simulink model "MVC2025_sim"  (R2024b)
settings: Solver=FixedStepAuto  StartTime=0.0  StopTime=Tsim  FixedStep=Ts
InitFcn:
  | warning('off','all')
StopFcn:
  | warning('on','all')
undefined symbols (not defined in the file or in its folder): BAT, BUS, CTRLpmsm, CTRLtug, CTRLves, DiscIntNeverNeededParam, ESM, GEN, magnitude, MOT, RLgain, SM, tau0, Ts, TUG, VES
libraries: fl_lib x47, nesl_utility x35, simulink x24, slpidlib x10, ee_lib x10, sdl_lib x3, rllib x1, batteryecm_lib x1
(part 1 of 3)
settings Model: Creator=andreaturno  LastModifiedBy=sirpd
settings OptimizationCC: ReuseModelBlockBuffer=off
settings DebuggingCC: UnconnectedInputMsg=warning  UnconnectedOutputMsg=warning  UnconnectedLineMsg=warning
settings ModelReferenceCC: EnableRefExpFcnMdlSchedulingChecks=on
settings RTWCC: GPUComputeCapability=3.5  DLArmComputeVersion=19.05

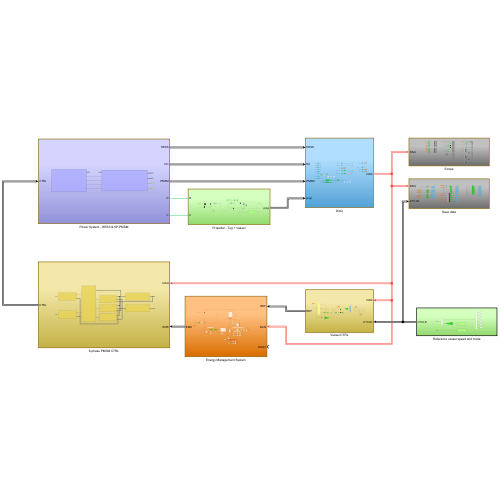
[thumbnail: Simulink's stored preview of the top-level diagram]
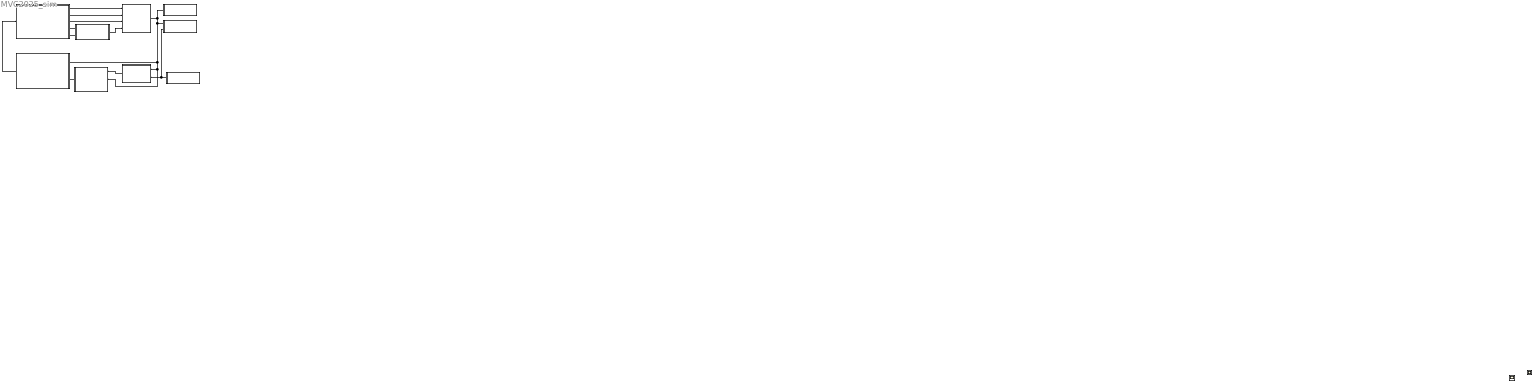
== system MVC2025_sim ==
  6-phase PMSM CTRL : Subsystem
  DAQ : Subsystem
  Energy Management System : Subsystem
  Power System - HESS & 6P-PMSM : Subsystem
  Propeller - Tug + Vessel : Subsystem
  Reference vessel speed and mode : Subsystem
  Save data : Subsystem
  Scope : Subsystem
  Vessel CTRL : Subsystem
  Scope1 : Scope
  Scope2 : Scope
  Scope3 : Scope
  wires:
  DAQ/1(DAQ) -> Save data/1(DAQ), Energy Management System/2(DAQ), Vessel CTRL/1(DAQ), 6-phase PMSM CTRL/1(DAQ), Scope/1(DAQ)
  Energy Management System/1(EMS) -> 6-phase PMSM CTRL/2(EMS)
  Power System - HESS & 6P-PMSM/1(HESS) -> DAQ/1(HESS)
  Power System - HESS & 6P-PMSM/2(DC) -> DAQ/2(DC)
  Power System - HESS & 6P-PMSM/3(PMSM) -> DAQ/3(PMSM)
  Propeller - Tug + Vessel/1(prop) -> DAQ/4(prop)
  Vessel CTRL/1(REF) -> Energy Management System/1(REF)
  Reference vessel speed and mode/1(CYCLE) -> Save data/2(CYCLE), Vessel CTRL/2(CYCLE)
  6-phase PMSM CTRL/1(CTRL) -> Power System - HESS & 6P-PMSM/1(CTRL)
  connections:
  Propeller - Tug + Vessel/LConn1 -- Power System - HESS & 6P-PMSM/RConn1
  Propeller - Tug + Vessel/LConn2 -- Power System - HESS & 6P-PMSM/RConn2

== system MVC2025_sim/6-phase PMSM CTRL ==
  In Bus Element : Inport  PortName=DAQ
  In Bus Element1 : Inport  Port=2  PortName=EMS
  "ABCDEF -> dqp-dqm-0z" : Subsystem
  "dq+-0z -> ABCDEF" : Subsystem
  duty cycles ABC : Subsystem
  duty cycles DEF : Subsystem
  i0z CTRL : Subsystem
  idq+ CTRL : Subsystem
  idq- CTRL : Subsystem
  reference currents : Subsystem
  Out Bus Element : Outport  PortName=CTRL  Element=SABC
  Out Bus Element1 : Outport  PortName=CTRL  Element=SDEF
  wires:
  In Bus Element/1 -> duty cycles ABC/2(DAQ), duty cycles DEF/2(DAQ), idq- CTRL/3(DAQ), "dq+-0z -> ABCDEF"/1(DAQ), idq+ CTRL/3(DAQ), "ABCDEF -> dqp-dqm-0z"/1(DAQ)
  "ABCDEF -> dqp-dqm-0z"/1(iSMPL) -> i0z CTRL/1(iSMPL), idq- CTRL/1(iSMPL), idq+ CTRL/1(iSMPL)
  reference currents/1(iSTAR) -> i0z CTRL/2(iSTAR), idq+ CTRL/2(iSTAR), idq- CTRL/2(iSTAR)
  duty cycles ABC/1(sABC) -> Out Bus Element/1
  duty cycles DEF/1(sABC) -> Out Bus Element1/1
  "dq+-0z -> ABCDEF"/1(vABC*) -> duty cycles ABC/1(VABC*)
  "dq+-0z -> ABCDEF"/2(vDEF*) -> duty cycles DEF/1(VDEF*)
  idq+ CTRL/1(vdq+*) -> "dq+-0z -> ABCDEF"/2(vdq+*)
  idq- CTRL/1(vdq-*) -> "dq+-0z -> ABCDEF"/3(vdq-*)
  i0z CTRL/1(v0z*) -> "dq+-0z -> ABCDEF"/4(v0z*)
  In Bus Element1/1 -> reference currents/1(EMS)

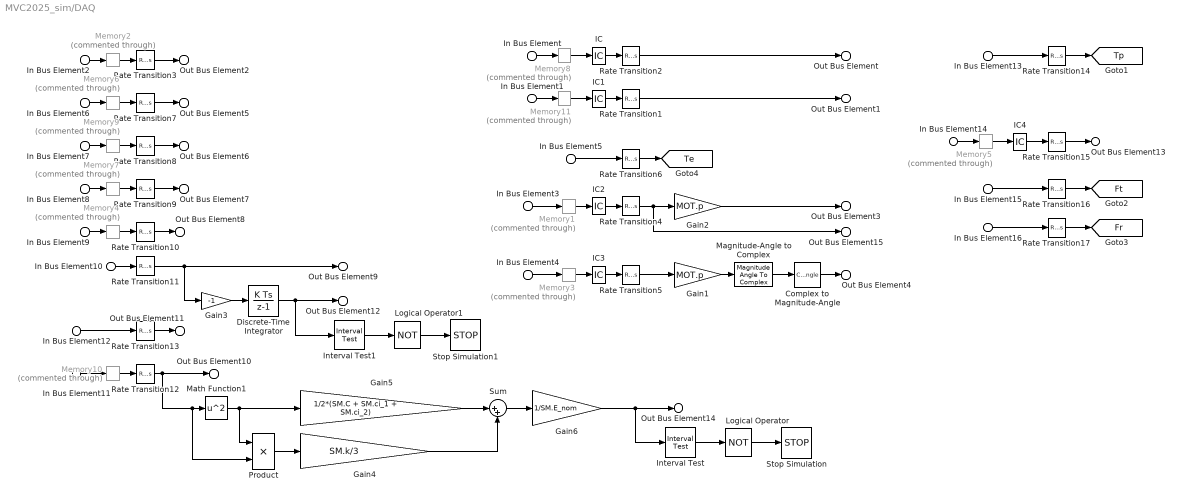
== system MVC2025_sim/DAQ ==
  In Bus Element9 : Inport  PortName=HESS  Element=vBP
  In Bus Element10 : Inport  PortName=HESS  Element=iBP
  In Bus Element11 : Inport  PortName=HESS  Element=vSM
  In Bus Element12 : Inport  PortName=HESS  Element=iSM
  In Bus Element2 : Inport  Port=2  PortName=DC  Element=vABC
  In Bus Element6 : Inport  Port=2  PortName=DC  Element=iABC
  In Bus Element7 : Inport  Port=2  PortName=DC  Element=vDEF
  In Bus Element8 : Inport  Port=2  PortName=DC  Element=iDEF
  In Bus Element : Inport  Port=3  PortName=PMSM  Element=iABC
  In Bus Element1 : Inport  Port=3  PortName=PMSM  Element=iDEF
  In Bus Element3 : Inport  Port=3  PortName=PMSM  Element=wm
  In Bus Element4 : Inport  Port=3  PortName=PMSM  Element=Om
  In Bus Element5 : Inport  Port=3  PortName=PMSM  Element=Te
  In Bus Element13 : Inport  Port=4  PortName=prop  Element=Tp
  In Bus Element14 : Inport  Port=4  PortName=prop  Element=V
  In Bus Element15 : Inport  Port=4  PortName=prop  Element=Ft
  In Bus Element16 : Inport  Port=4  PortName=prop  Element=Fr
  Complex to Magnitude-Angle : ComplexToMagnitudeAngle  Output=Angle
  Discrete-Time Integrator : DiscreteIntegrator  gainval=1/BAT.Q_nom  InitialCondition=BAT.SoC_0  SampleTime=Ts  ICPrevOutput=DiscIntNeverNeededParam  ICPrevScaledInput=DiscIntNeverNeededParam
  Gain1 : Gain  Gain=MOT.p
  Gain2 : Gain  Gain=MOT.p
  Gain3 : Gain  Gain=-1
  Gain4 : Gain  Gain=SM.k/3
  Gain5 : Gain  Gain=1/2*(SM.C + SM.ci_1 + SM.ci_2)
  Gain6 : Gain  Gain=1/SM.E_nom
  IC{,1..4} (5 alike) : InitialCondition  Value=0
  Interval Test : simulink/Logic and Bit Operations/Interval Test  IntervalClosedRight=on  uplimit=SM.SoE_max  IntervalClosedLeft=on  lowlimit=SM.SoE_min  OutDataTypeStr=boolean
  Interval Test1 : simulink/Logic and Bit Operations/Interval Test  IntervalClosedRight=on  uplimit=BAT.SoC_max+1e-7  IntervalClosedLeft=on  lowlimit=BAT.SoC_min  OutDataTypeStr=boolean
  Logical Operator : Logic  Operator=NOT  AllPortsSameDT=off  OutDataTypeStr=boolean
  Logical Operator1 : Logic  Operator=NOT  AllPortsSameDT=off  OutDataTypeStr=boolean
  Magnitude-Angle to Complex : MagnitudeAngleToComplex  Input=Angle  ConstantPart=1
  Math Function1 : Math  Operator=square
  Memory{1,3,8,10..11} (5 alike) : Memory  Commented=through  InitialCondition=SM.V_0
  Memory2 : Memory  Commented=through  InitialCondition=BUS.Vdc
  Memory{4..7} (4 alike) : Memory  Commented=through
  Memory9 : Memory  Commented=through  InitialCondition=BUS.Vdc
  Product : Product
  Rate Transition{1..2,4..5} (4 alike) : RateTransition  Integrity=off  Deterministic=off  OutPortSampleTime=Ts
  Rate Transition10 : RateTransition  InitialCondition=BAT.V_nom  OutPortSampleTime=Ts
  Rate Transition{6,11,13,16..17} (5 alike) : RateTransition  OutPortSampleTime=Ts
  Rate Transition12 : RateTransition  InitialCondition=SM.V_0  OutPortSampleTime=Ts
  Rate Transition{3,7..9,14..15} (6 alike) : RateTransition  Integrity=off  OutPortSampleTime=Ts
  Stop Simulation : Stop
  Stop Simulation1 : Stop
  Sum : Sum  Inputs=|++
  Out Bus Element : Outport  PortName=DAQ  Element=iABC
  Out Bus Element1 : Outport  PortName=DAQ  Element=iDEF
  Out Bus Element2 : Outport  PortName=DAQ  Element=VDC_ABC
  Out Bus Element3 : Outport  PortName=DAQ  Element=w
  Out Bus Element4 : Outport  PortName=DAQ  Element=O
  Out Bus Element5 : Outport  PortName=DAQ  Element=iDC_ABC
  Out Bus Element6 : Outport  PortName=DAQ  Element=VDC_DEF
  Out Bus Element7 : Outport  PortName=DAQ  Element=iDC_DEF
  Out Bus Element8 : Outport  PortName=DAQ  Element=vBP
  Out Bus Element9 : Outport  PortName=DAQ  Element=iBP
  Out Bus Element10 : Outport  PortName=DAQ  Element=vSM
  Out Bus Element11 : Outport  PortName=DAQ  Element=iSM
  Out Bus Element13 : Outport  PortName=DAQ  Element=V
  Out Bus Element12 : Outport  PortName=DAQ  Element=SoC_BP
  Out Bus Element14 : Outport  PortName=DAQ  Element=SoE_SM
  Out Bus Element15 : Outport  PortName=DAQ  Element=wm
  tag scope: Fr=global, Ft=global, Te=global, Tp=global
  wires:
  Rate Transition2/1 -> Out Bus Element/1
  Rate Transition1/1 -> Out Bus Element1/1
  In Bus Element2/1 -> Memory2/1
  Rate Transition4/1 -> Out Bus Element15/1, Gain2/1
  Gain2/1 -> Out Bus Element3/1
  In Bus Element4/1 -> Memory3/1
  Rate Transition5/1 -> Gain1/1
  Gain1/1 -> Magnitude-Angle to Complex/1
  Complex to Magnitude-Angle/1 -> Out Bus Element4/1
  Magnitude-Angle to Complex/1 -> Complex to Magnitude-Angle/1
  In Bus Element/1 -> Memory8/1
  In Bus Element1/1 -> Memory11/1
  Memory2/1 -> Rate Transition3/1
  In Bus Element3/1 -> Memory1/1
  In Bus Element5/1 -> Rate Transition6/1
  Rate Transition6/1 -> [Te]
  IC/1 -> Rate Transition2/1
  Memory6/1 -> Rate Transition7/1
  Rate Transition7/1 -> Out Bus Element5/1
  In Bus Element6/1 -> Memory6/1
  Rate Transition9/1 -> Out Bus Element7/1
  In Bus Element8/1 -> Memory7/1
  In Bus Element7/1 -> Memory9/1
  Rate Transition8/1 -> Out Bus Element6/1
  In Bus Element9/1 -> Memory4/1
  Rate Transition10/1 -> Out Bus Element8/1
  Rate Transition11/1 -> Gain3/1, Out Bus Element9/1
  In Bus Element10/1 -> Rate Transition11/1
  In Bus Element12/1 -> Rate Transition13/1
  Rate Transition13/1 -> Out Bus Element11/1
  Rate Transition12/1 -> Product/2, Math Function1/1, Out Bus Element10/1
  In Bus Element14/1 -> Memory5/1
  Rate Transition15/1 -> Out Bus Element13/1
  IC4/1 -> Rate Transition15/1
  In Bus Element15/1 -> Rate Transition16/1
  Rate Transition16/1 -> [Ft]
  Rate Transition17/1 -> [Fr]
  In Bus Element16/1 -> Rate Transition17/1
  Memory7/1 -> Rate Transition9/1
  Memory9/1 -> Rate Transition8/1
  In Bus Element13/1 -> Rate Transition14/1
  Rate Transition14/1 -> [Tp]
  Gain3/1 -> Discrete-Time Integrator/1
  Product/1 -> Gain4/1
  Math Function1/1 -> Gain5/1, Product/1
  Gain5/1 -> Sum/1
  Gain4/1 -> Sum/2
  Sum/1 -> Gain6/1
  In Bus Element11/1 -> Memory10/1
  Rate Transition3/1 -> Out Bus Element2/1
  Memory10/1 -> Rate Transition12/1
  IC1/1 -> Rate Transition1/1
  IC2/1 -> Rate Transition4/1
  IC3/1 -> Rate Transition5/1
  Memory1/1 -> IC2/1
  Memory3/1 -> IC3/1
  Memory4/1 -> Rate Transition10/1
  Memory5/1 -> IC4/1
  Memory8/1 -> IC/1
  Memory11/1 -> IC1/1
  Logical Operator1/1 -> Stop Simulation1/1
  Interval Test1/1 -> Logical Operator1/1
  Discrete-Time Integrator/1 -> Out Bus Element12/1, Interval Test1/1
  Logical Operator/1 -> Stop Simulation/1
  Interval Test/1 -> Logical Operator/1
  Gain6/1 -> Interval Test/1, Out Bus Element14/1

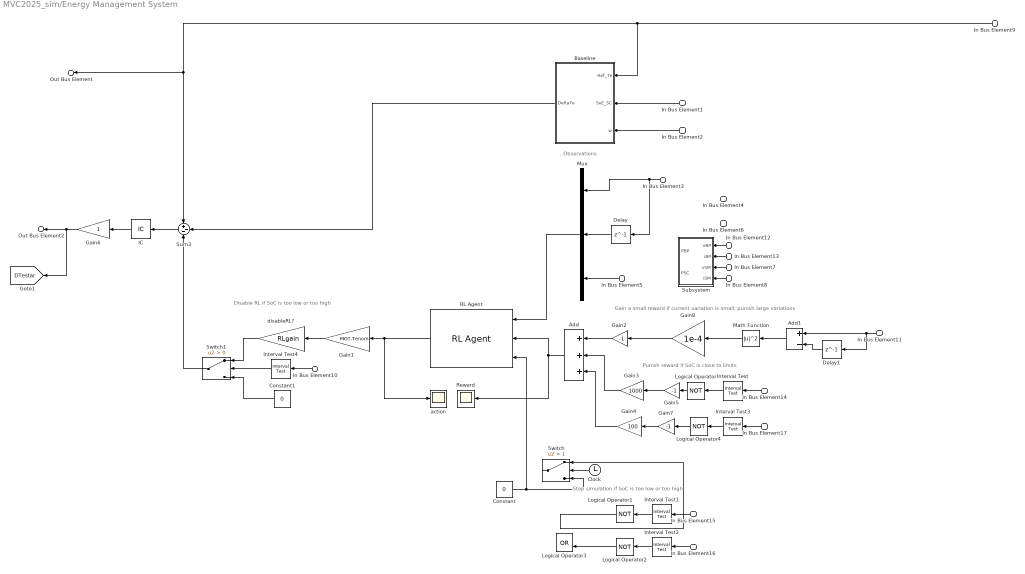
== system MVC2025_sim/Energy Management System ==
  note: Disable RL if SoC is too low or too high
  note: Punish reward if SoC is close to limits
  note: Gain a small reward if current variation is small; punish large variations
  note: Observations
  note: Stop simulation if SoC is too low or too high
  In Bus Element9 : Inport  PortName=REF  Element=Te
  In Bus Element6 : Inport  PortName=REF  Element=Te
  In Bus Element{1,5,10,14} (4 alike) : Inport  Port=2  PortName=DAQ  Element=SoE_SM
  In Bus Element2 : Inport  Port=2  PortName=DAQ  Element=w
  In Bus Element3 : Inport  Port=2  PortName=DAQ  Element=iBP
  In Bus Element13 : Inport  Port=2  PortName=DAQ  Element=iBP
  In Bus Element11 : Inport  Port=2  PortName=DAQ  Element=iBP
  In Bus Element4 : Inport  Port=2  PortName=DAQ  Element=SoC_BP
  In Bus Element16 : Inport  Port=2  PortName=DAQ  Element=SoC_BP
  In Bus Element17 : Inport  Port=2  PortName=DAQ  Element=SoC_BP
  In Bus Element12 : Inport  Port=2  PortName=DAQ  Element=vBP
  In Bus Element7 : Inport  Port=2  PortName=DAQ  Element=vSM
  In Bus Element8 : Inport  Port=2  PortName=DAQ  Element=iSM
  In Bus Element15 : Inport  Port=3  PortName=DAQ1  Element=SoE_SM
  Add : Sum  Inputs=+++
  Add1 : Sum  Inputs=+-
  Baseline : Subsystem
  Clock : Clock
  Constant : Constant  Value=0
  Constant1 : Constant  Value=0
  Delay : Delay  DelayLength=1  SampleTime=Ts
  Delay1 : Delay  DelayLength=1  SampleTime=Ts
  Gain1 : Gain  Gain=MOT.Tenom
  Gain2 : Gain  Gain=-1
  Gain3 : Gain  Gain=1000
  Gain4 : Gain  Gain=100
  Gain5 : Gain  Gain=-1
  Gain6 : Gain
  Gain7 : Gain  Gain=-1
  Gain8 : Gain  Gain=1e-4
  IC : InitialCondition  Value=0
  Interval Test : simulink/Logic and Bit Operations/Interval Test  IntervalClosedRight=on  uplimit=0.95  IntervalClosedLeft=on  lowlimit=0.05  OutDataTypeStr=boolean
  Interval Test1 : simulink/Logic and Bit Operations/Interval Test  IntervalClosedRight=on  uplimit=0.99  IntervalClosedLeft=on  lowlimit=0.01  OutDataTypeStr=boolean
  Interval Test2 : simulink/Logic and Bit Operations/Interval Test  IntervalClosedRight=on  uplimit=0.99  IntervalClosedLeft=on  lowlimit=0.01  OutDataTypeStr=boolean
  Interval Test3 : simulink/Logic and Bit Operations/Interval Test  IntervalClosedRight=on  uplimit=0.99  IntervalClosedLeft=on  lowlimit=0.01  OutDataTypeStr=boolean
  Interval Test4 : simulink/Logic and Bit Operations/Interval Test  IntervalClosedRight=on  uplimit=0.55  IntervalClosedLeft=on  lowlimit=0.03  OutDataTypeStr=boolean
  Logical Operator{,1..2,4} (4 alike) : Logic  Operator=NOT  AllPortsSameDT=off  OutDataTypeStr=boolean
  Logical Operator3 : Logic  Operator=OR  AllPortsSameDT=off  OutDataTypeStr=boolean
  Math Function : Math  Operator=magnitude^2
  Mux : Mux  Inputs=3
  RL Agent : rllib/RL Agent  Agent=agent  ExternalActionAsInput=off  ProvideLastAction=off  ProvideCumRwd=off  TreatAsDirectFeedthrough=on  UseStrictObservationDataTypes=off
  Reward : Scope
  Subsystem : Subsystem
  Sum3 : Sum  Inputs=+--
  Switch : Switch  Criteria=u2 > Threshold  Threshold=1  SaturateOnIntegerOverflow=off  InputSameDT=off
  Switch1 : Switch  Criteria=u2 > Threshold  SaturateOnIntegerOverflow=off  InputSameDT=off
  action : Scope
  disableRL? : Gain  Gain=RLgain
  Out Bus Element : Outport  PortName=EMS  Element=Te
  Out Bus Element2 : Outport  PortName=EMS  Element=DTe
  tag scope: DTestar=global
  wires:
  In Bus Element9/1 -> Sum3/1, Out Bus Element/1, Baseline/1(Ref_Te)
  Sum3/1 -> IC/1
  IC/1 -> Gain6/1
  Gain6/1 -> Out Bus Element2/1, [DTestar]
  In Bus Element1/1 -> Baseline/2(SoE_SC)
  In Bus Element2/1 -> Baseline/3(w)
  Baseline/1(DeltaTe) -> Sum3/2
  Gain1/1 -> disableRL?/1
  Add/1 -> RL Agent/2, Reward/1
  Mux/1 -> RL Agent/1
  In Bus Element3/1 -> Delay/1, Mux/1
  In Bus Element12/1 -> Subsystem/1(vBP)
  In Bus Element13/1 -> Subsystem/2(iBP)
  In Bus Element7/1 -> Subsystem/3(vSM)
  In Bus Element8/1 -> Subsystem/4(iSM)
  Add1/1 -> Math Function/1
  Math Function/1 -> Gain8/1
  In Bus Element14/1 -> Interval Test/1
  Interval Test/1 -> Logical Operator/1
  Gain3/1 -> Add/2
  Interval Test1/1 -> Logical Operator1/1
  In Bus Element15/1 -> Interval Test1/1
  Interval Test2/1 -> Logical Operator2/1
  In Bus Element16/1 -> Interval Test2/1
  Logical Operator2/1 -> Logical Operator3/2
  Interval Test3/1 -> Logical Operator4/1
  In Bus Element17/1 -> Interval Test3/1
  Gain4/1 -> Add/3
  Gain5/1 -> Gain3/1
  Logical Operator/1 -> Gain5/1
  Logical Operator4/1 -> Gain7/1
  Gain7/1 -> Gain4/1
  RL Agent/1 -> action/1, Gain1/1
  Logical Operator1/1 -> Switch/1
  Clock/1 -> Switch/2
  Constant/1 -> RL Agent/3, Switch/3
  Gain2/1 -> Add/1
  Gain8/1 -> Gain2/1
  In Bus Element5/1 -> Mux/3
  Delay/1 -> Mux/2
  In Bus Element11/1 -> Delay1/1, Add1/1
  Delay1/1 -> Add1/2
  In Bus Element10/1 -> Interval Test4/1
  Interval Test4/1 -> Switch1/2
  disableRL?/1 -> Switch1/1
  Constant1/1 -> Switch1/3
  Switch1/1 -> Sum3/3

== system MVC2025_sim/Power System - HESS & 6P-PMSM ==
  In Bus Element : Inport  PortName=CTRL
  6-phase PMSM drive : Subsystem
  Hybrid Energy Storage System (HESS) : Subsystem
  R : PMIOPort  Side=Right
  C : PMIOPort  Port=2  Side=Right
  Out Bus Element2 : Outport  PortName=HESS
  Out Bus Element14 : Outport  Port=2  PortName=DC
  Out Bus Element1 : Outport  Port=3  PortName=PMSM
  wires:
  6-phase PMSM drive/1(DC) -> Out Bus Element14/1
  Hybrid Energy Storage System (HESS)/1(HESS) -> Out Bus Element2/1
  In Bus Element/1 -> 6-phase PMSM drive/1(CTRL)
  6-phase PMSM drive/2(PMSM) -> Out Bus Element1/1
  connections:
  Hybrid Energy Storage System (HESS)/RConn1 -- 6-phase PMSM drive/LConn1
  Hybrid Energy Storage System (HESS)/RConn2 -- 6-phase PMSM drive/LConn2
  Hybrid Energy Storage System (HESS)/RConn3 -- 6-phase PMSM drive/LConn3
  Hybrid Energy Storage System (HESS)/RConn4 -- 6-phase PMSM drive/LConn4
  R/RConn1 -- 6-phase PMSM drive/RConn1
  C/RConn1 -- 6-phase PMSM drive/RConn2

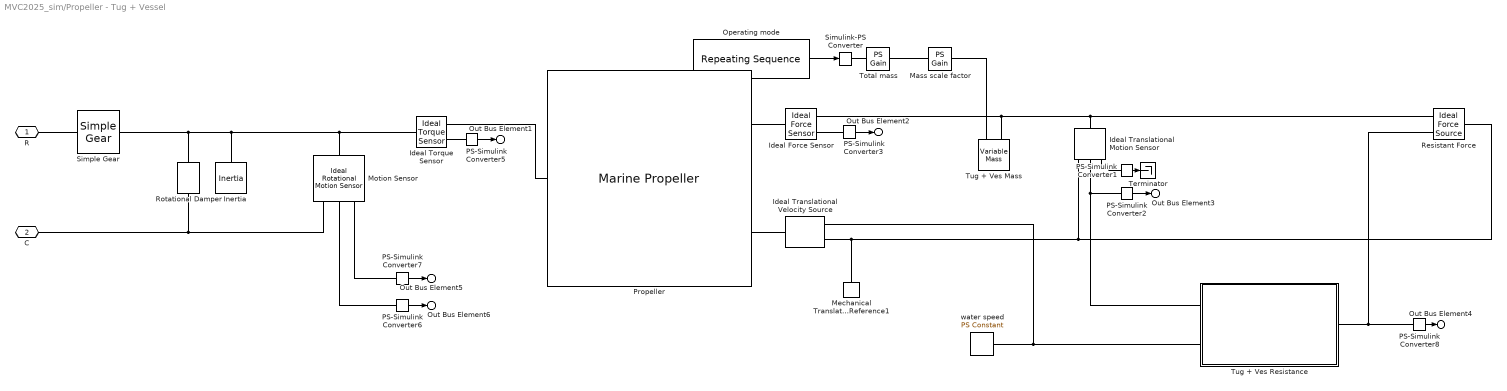
== system MVC2025_sim/Propeller - Tug + Vessel ==
  Ideal Force Sensor : fl_lib/Mechanical/Mechanical Sensors/Ideal Force Sensor
  Ideal Torque Sensor : fl_lib/Mechanical/Mechanical Sensors/Ideal Torque Sensor
  Ideal Translational Motion Sensor : fl_lib/Mechanical/Mechanical Sensors/Ideal Translational Motion Sensor  reference=foundation.enum.MeasurementReference.difference  acceleration_port=false  velocity_port=true  position_port=true  offset=0 m
  Ideal Translational Velocity Source : fl_lib/Mechanical/Mechanical Sources/Ideal Translational Velocity Source
  Inertia : fl_lib/Mechanical/Rotational Elements/Inertia  inertia=TUG.Jp kg*m^2  num_ports=foundation.enum.numPorts2.one  w_specify=off  w_priority=High  w=0 rad/s  w_nominal_specify=off  w_nominal_value=1  w_nominal_unit=rad/s  t_specify=off  t_priority=None  t=0 N*m  t_nominal_specify=off  t_nominal_value=1  t_nominal_unit=N*m
  Mass scale factor : fl_lib/Physical Signals/Functions/PS Gain  gain=0.5
  Mechanical Translational Reference1 : fl_lib/Mechanical/Translational Elements/Mechanical Translational Reference
  Motion Sensor : fl_lib/Mechanical/Mechanical Sensors/Ideal Rotational Motion Sensor  reference=foundation.enum.MeasurementReference.difference  acceleration_port=false  velocity_port=true  position_port=true  wrap_angle=simscape.enum.onoff.off  offset=0 rad
  Operating mode : simulink/Sources/Repeating Sequence  rep_seq_t=V_star.time  rep_seq_y=V_star.mode
  PS-Simulink Converter1 : nesl_utility/PS-Simulink Converter  PhysicalDomain=network_engine_domain  SubClassName=ps_output  LeftPortType=input  RightPortType=output  PseudoPeriodic=off  Frequencies=[]  VectorFormat=1-D array  Unit=inherit  AffineConversion=off
  PS-Simulink Converter2 : nesl_utility/PS-Simulink Converter  PhysicalDomain=network_engine_domain  SubClassName=ps_output  LeftPortType=input  RightPortType=output  PseudoPeriodic=off  Frequencies=[]  VectorFormat=1-D array  Unit=inherit  AffineConversion=off
  PS-Simulink Converter3 : nesl_utility/PS-Simulink Converter  PhysicalDomain=network_engine_domain  SubClassName=ps_output  LeftPortType=input  RightPortType=output  PseudoPeriodic=off  Frequencies=[]  VectorFormat=1-D array  Unit=N  AffineConversion=off
  PS-Simulink Converter5 : nesl_utility/PS-Simulink Converter  PhysicalDomain=network_engine_domain  SubClassName=ps_output  LeftPortType=input  RightPortType=output  PseudoPeriodic=off  Frequencies=[]  VectorFormat=1-D array  Unit=N*m  AffineConversion=off
  PS-Simulink Converter6 : nesl_utility/PS-Simulink Converter  PhysicalDomain=network_engine_domain  SubClassName=ps_output  LeftPortType=input  RightPortType=output  PseudoPeriodic=off  Frequencies=[]  VectorFormat=1-D array  Unit=rad/s  AffineConversion=off
  PS-Simulink Converter7 : nesl_utility/PS-Simulink Converter  PhysicalDomain=network_engine_domain  SubClassName=ps_output  LeftPortType=input  RightPortType=output  PseudoPeriodic=off  Frequencies=[]  VectorFormat=1-D array  Unit=rad  AffineConversion=off
  PS-Simulink Converter8 : nesl_utility/PS-Simulink Converter  PhysicalDomain=network_engine_domain  SubClassName=ps_output  LeftPortType=input  RightPortType=output  PseudoPeriodic=off  Frequencies=[]  VectorFormat=1-D array  Unit=inherit  AffineConversion=off
  Propeller : sdl_lib/Engines & Motors/Marine Propeller  parameterization=sdl.enum.PropellerParameterization.Constant  pitch_type=foundation.enum.constant_controlled.constant  direction=sdl.enum.PropellerDirection.Positive  D=TUG.Dm m  kt_const=TUG.kT  kq_const=TUG.kQ  kt_poly_fixed=[.063, -.19, -.25, .37]  kq_poly_fixed=[.0043, -.021, -.03, .05]  pitch_ratio_TLU=[-.5, .5, .7, .9, 1.1, 1.4]  kt_poly_TLU=[.04, -.1, -.24, .12; .118, -.24, -.24, .19; .082, -.21, -.25, .28; .063, -.19, -.25, .37; .055, -.17, -.25, .45; .064, -.21, -.19, .55]  kq_poly_TLU=[.02, -.06, -.02, .02; .04, -.034, -.016, .018; .0076, -.02, -.023, .031; .0043, -.021, -.03, .05; .0047, -.024, -.036, .073; .0045, -.025, -.044, .11]  J_tab_TLU=[0, .3, .5, .7, .9, 1.2, 1.5]  kt_tab_fixed=[.37, .28, .21, .12, .033, -.098, -.23]  kq_tab_fixed=[.049, .039, .03, .02, .0096, -.0093, -.028]  kt_tab_TLU=[.12, .04, -.02, -.083, -.15, -.24, -.33; .19, .1, .029, -.047, -.12, -.23, -.35; .28, .19, .12, .032, -.054, -.18, -.31; .37, .28, .21, .12, .033, -.098, -.23; .45, .36, .29, .21, .13, -.0057, -.16; .54, .47, .41, .33, .25, .13, .0029]  kq_tab_TLU=[.02, .0091, -.0025, -.017, -.032, -.056, -.078; .017, .011, .006, .0009, -.0041, -.012, -.019; .03, .022, .015, .0074, -.0008, -.013, -.026; .049, .039, .03, .02, .0096, -.0093, -.028; .072, .06, .05, .038, .025, .0042, -.015; .11, .097, .085, .071, .057, .033, .0065]  beta_TLU=linspace(0, 360, 10) deg  Ct_TLU_1D=0.2 * sind(linspace(0, 360, 10) - 200)  Cq_TLU_1D=0.015 * sind(linspace(0, 360, 10) - 200)  Ct_TLU_2D=[0.15 * sind(linspace(0, 360, 10) - 200); 0.20 * sind(linspace(0, 360, 10) - 200); 0.25 * sind(linspace(0, 360, 10) - 200); 0.30 * sind(linspace(0, 360, 10) - 200); 0.35 * sind(linspace(0, 360, 10) - 200); 0.40 * sind(linspace(0, 360, 10) - 200)]  Cq_TLU_2D=[0.010 * sind(linspace(0, 360, 10) - 200); 0.015 * sind(linspace(0, 360, 10) - 200); 0.020 * sind(linspace(0, 360, 10) - 200); 0.025 * sind(linspace(0, 360, 10) - 200); 0.030 * sind(linspace(0, 360, 10) - 200); 0.035 * sind(linspace(0, 360, 10) - 200)]  interp_method=simscape.enum.interpolation.linear  extrap_method=simscape.enum.extrapolation.linear  density_spec=foundation.enum.constant_variable.constant  rho=GEN.rhow kg/m^3  rotational_ports=sdl.enum.ConnectionType.Conserving  translational_ports=sdl.enum.ConnectionType.Conserving  wake_fraction=TUG.wf  model_inertia=false  propeller_inertia=0.1 kg*m^2  propeller_mass=10 kg  efficiency_sensor=simscape.enum.onoff.off  n_thr=0.001 Hz  k_thr=0.001  operation_check=simscape.enum.assert.action.warn  expose_port_C=0  w_specify=off  w_priority=None  w=0 rad/s  w_nominal_specify=off  w_nominal_value=1  w_nominal_unit=rad/s  Q_specify=off  Q_priority=None  Q=0 N*m  Q_nominal_specify=off  Q_nominal_value=1  Q_nominal_unit=N*m  v_specify=off  v_priority=None  v=0 m/s  v_nominal_specify=off  v_nominal_value=1  v_nominal_unit=m/s  thrust_specify=off  thrust_priority=None  thrust=0 N  thrust_nominal_specify=off  thrust_nominal_value=1  thrust_nominal_unit=N
      settings: InternalSimscapePortConfiguration="{\"Bottom\":[],\"Left\":[{\"id\":\"R1\",\"label\":\"R1\",\"type\":\"foundation.mechanical.rotational.rotational\"}],\"Right\":[{\"id\":\"R2\",\"label\":\"R2\",\"type\":\"foundation.mechanical.translational.translational\"},{\"id\":\"C2\",\"label\":\"C2\",\"type\":\"foundation.mechanical.translational.translational\"}],\"Top\":[]}"
  Resistant Force : fl_lib/Mechanical/Mechanical Sources/Ideal Force Source
  Rotational Damper : fl_lib/Mechanical/Rotational Elements/Rotational Damper  D=TUG.Dp N*m/(rad/s)  w_specify=off  w_priority=None  w=0 rad/s  w_nominal_specify=off  w_nominal_value=1  w_nominal_unit=rad/s  t_specify=off  t_priority=None  t=0 N*m  t_nominal_specify=off  t_nominal_value=1  t_nominal_unit=N*m
  Simple Gear : sdl_lib/Gears/Simple Gear  ratio=1/TUG.tau  rotation_direction=sdl.enum.shaftOutputDirection.same  friction_model=sdl.enum.gear_efficiencies_load.off  T_noload=0.1 N*m  T_nom=5 N*m  efficiency_nom=0.8  efficiency=0.8  temperature_TLU=[280, 300, 320] K  load_TLU=[1, 5, 10] N*m  efficiency_TLU=[.95, .9, .85]  efficiency_TLU2=[.85, .8, .75; .95, .9, .85; .85, .8, .7]  w_thr=0.01 rad/s  pwr_thr=0.001 W  enable_backlash=false  hardstop_model=simscape.enum.hardstop.smooth  backlash_distance=1e-3 mm  r_base=0.1 m  transition=1e-4 mm  backlash_stiffness=1e7 N/m  backlash_damping=1e6 N*s/m  coeff_rest=0  v_tol=0.001 m/s  f_tol=0 N  mu_visc=[0, 0] N*m*s/rad  thermal_mass=50 J/K  temperature_specify=off  temperature_priority=High  temperature=300 K  temperature_nominal_specify=off  temperature_nominal_value=1  temperature_nominal_unit=K  x_backlash_specify=off  x_backlash_priority=None  x_backlash=0 mm  x_backlash_nominal_specify=off  x_backlash_nominal_value=1  x_backlash_nominal_unit=mm  f_hardstop_specify=off  f_hardstop_priority=None  f_hardstop=0 N  f_hardstop_nominal_specify=off  f_hardstop_nominal_value=1  f_hardstop_nominal_unit=N  v_backlash_specify=off  v_backlash_priority=None  v_backlash=0 m/s  v_backlash_nominal_specify=off  v_backlash_nominal_value=1  v_backlash_nominal_unit=m/s
  Simulink-PS Converter : nesl_utility/Simulink-PS Converter  PhysicalDomain=network_engine_domain  SubClassName=ps_input  LeftPortType=input  RightPortType=output  PseudoPeriodic=off  Frequencies=[]  NoiseDistribution=none  NoiseParameters=[]  Unit=1  AffineConversion=off  FilteringAndDerivatives=provide  SimscapeFilterOrder=1  InputFilterTimeConstant=0.001  UdotUserProvided=0
  Terminator : Terminator
  Total mass : fl_lib/Physical Signals/Functions/PS Gain  gain=(TUG.M + VES.M) kg
  Tug + Ves Mass : sdl_lib/Inertias & Loads/Variable Mass  minimum_mass=TUG.M kg  p_specify=off  p_priority=High  p=0 kg*m/s  p_nominal_specify=off  p_nominal_value=1  p_nominal_unit=kg*m/s
      settings: InternalSimscapePortConfiguration="{\"Bottom\":[],\"Left\":[{\"id\":\"M\",\"label\":\"\",\"type\":\"input\"},{\"id\":\"A\",\"label\":\"\",\"type\":\"foundation.mechanical.translational.translational\"}],\"Right\":[],\"Top\":[]}"
  Tug + Ves Resistance : Subsystem
  water speed : fl_lib/Physical Signals/Sources/PS Constant  constant=TUG.Vw m/s
  R : PMIOPort  Side=Left
  C : PMIOPort  Port=2  Side=Left
  Out Bus Element3 : Outport  PortName=prop  Element=V
  Out Bus Element1 : Outport  PortName=prop  Element=Tp
  Out Bus Element2 : Outport  PortName=prop  Element=Ft
  Out Bus Element4 : Outport  PortName=prop  Element=Fr
  Out Bus Element5 : Outport  PortName=prop  Element=Op
  Out Bus Element6 : Outport  PortName=prop  Element=Wp
  wires:
  PS-Simulink Converter1/1 -> Terminator/1
  PS-Simulink Converter2/1 -> Out Bus Element3/1
  PS-Simulink Converter5/1 -> Out Bus Element1/1
  PS-Simulink Converter3/1 -> Out Bus Element2/1
  PS-Simulink Converter7/1 -> Out Bus Element5/1
  PS-Simulink Converter6/1 -> Out Bus Element6/1
  PS-Simulink Converter8/1 -> Out Bus Element4/1
  Operating mode/1 -> Simulink-PS Converter/1
  connections:
  Propeller/LConn1 -- Ideal Torque Sensor/RConn1
  C/RConn1 -- Rotational Damper/RConn1 -- Motion Sensor/RConn1
  Ideal Translational Velocity Source/LConn1 -- Propeller/RConn2
  Ideal Translational Motion Sensor/LConn1 -- Ideal Force Sensor/RConn1 -- Tug + Ves Mass/LConn2 -- Resistant Force/RConn2
  Mechanical Translational Reference1/LConn1 -- Resistant Force/LConn1 -- Ideal Translational Motion Sensor/RConn1 -- Ideal Translational Velocity Source/RConn2
  PS-Simulink Converter1/LConn1 -- Ideal Translational Motion Sensor/RConn3
  Ideal Torque Sensor/LConn1 -- Motion Sensor/LConn1 -- Inertia/LConn1 -- Simple Gear/LConn1 -- Rotational Damper/LConn1
  PS-Simulink Converter5/LConn1 -- Ideal Torque Sensor/RConn2
  PS-Simulink Converter3/LConn1 -- Ideal Force Sensor/RConn2
  Ideal Force Sensor/LConn1 -- Propeller/RConn1
  Simple Gear/RConn1 -- R/RConn1
  Motion Sensor/RConn2 -- PS-Simulink Converter6/LConn1
  Motion Sensor/RConn3 -- PS-Simulink Converter7/LConn1
  Simulink-PS Converter/RConn1 -- Total mass/LConn1
  Total mass/RConn1 -- Mass scale factor/LConn1
  Mass scale factor/RConn1 -- Tug + Ves Mass/LConn1
  Tug + Ves Resistance/RConn1 -- PS-Simulink Converter8/LConn1 -- Resistant Force/RConn1
  Ideal Translational Motion Sensor/RConn2 -- Tug + Ves Resistance/LConn1 -- PS-Simulink Converter2/LConn1
  water speed/RConn1 -- Tug + Ves Resistance/LConn2 -- Ideal Translational Velocity Source/RConn1

== system MVC2025_sim/Reference vessel speed and mode ==
  Manual Switch : ManualSwitch  CurrentSetting=0
  Operating mode : simulink/Sources/Repeating Sequence  rep_seq_t=V_star.time  rep_seq_y=V_star.mode
  Speed profile [kts] : simulink/Sources/Repeating Sequence  rep_seq_t=V_star.time  rep_seq_y=V_star.speed_kts
  Sum : Sum  Inputs=6
  Vref#00 : simulink/Sources/Ramp  slope=TUG.Vn/2  start=0  InitialOutput=0
  Vref#01 : simulink/Sources/Ramp  slope=-TUG.Vn/2  start=1  InitialOutput=0
  Vref#02 : simulink/Sources/Ramp  slope=-TUG.Vn/2/7  start=3  InitialOutput=0
  Vref#03 : simulink/Sources/Ramp  slope=TUG.Vn/2/7  start=10  InitialOutput=0
  Vref#04 : simulink/Sources/Ramp  slope=TUG.Vn/1  start=15  InitialOutput=0
  Vref#05 : simulink/Sources/Ramp  slope=-TUG.Vn/1  start=16  InitialOutput=0
  kts to m/s : Gain  Gain=0.514444
  Out Bus Element : Outport  PortName=CYCLE  Element=V_star
  Out Bus Element1 : Outport  PortName=CYCLE  Element=mode
  wires:
  Vref#00/1 -> Sum/1
  Vref#01/1 -> Sum/2
  Vref#02/1 -> Sum/3
  Vref#03/1 -> Sum/4
  Vref#04/1 -> Sum/5
  Vref#05/1 -> Sum/6
  Manual Switch/1 -> Out Bus Element/1
  Sum/1 -> Manual Switch/1
  kts to m/s/1 -> Manual Switch/2
  Speed profile [kts]/1 -> kts to m/s/1
  Operating mode/1 -> Out Bus Element1/1

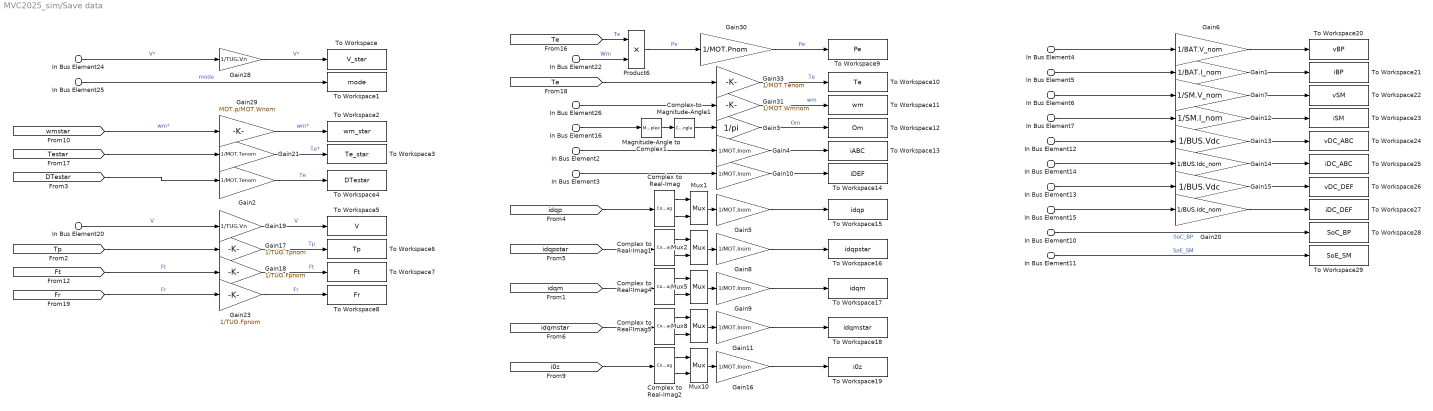
== system MVC2025_sim/Save data ==
  In Bus Element16 : Inport  PortName=DAQ  Element=O
  In Bus Element2 : Inport  PortName=DAQ  Element=iABC
  In Bus Element3 : Inport  PortName=DAQ  Element=iDEF
  In Bus Element4 : Inport  PortName=DAQ  Element=vBP
  In Bus Element5 : Inport  PortName=DAQ  Element=iBP
  In Bus Element6 : Inport  PortName=DAQ  Element=vSM
  In Bus Element7 : Inport  PortName=DAQ  Element=iSM
  In Bus Element20 : Inport  PortName=DAQ  Element=V
  In Bus Element10 : Inport  PortName=DAQ  Element=SoC_BP
  In Bus Element11 : Inport  PortName=DAQ  Element=SoE_SM
  In Bus Element26 : Inport  PortName=DAQ  Element=wm
  In Bus Element22 : Inport  PortName=DAQ  Element=wm
  In Bus Element12 : Inport  PortName=DAQ  Element=VDC_ABC
  In Bus Element13 : Inport  PortName=DAQ  Element=VDC_DEF
  In Bus Element14 : Inport  PortName=DAQ  Element=iDC_ABC
  In Bus Element15 : Inport  PortName=DAQ  Element=iDC_DEF
  In Bus Element24 : Inport  Port=2  PortName=CYCLE  Element=V_star
  In Bus Element25 : Inport  Port=2  PortName=CYCLE  Element=mode
  Complex to Real-Imag{,1..2,4..5} (5 alike) : ComplexToRealImag
  Complex to Magnitude-Angle1 : ComplexToMagnitudeAngle  Output=Angle
  Gain1 : Gain  Gain=1/BAT.I_nom
  Gain{4..5,8..11,16} (7 alike) : Gain  Gain=1/MOT.Inom
  Gain12 : Gain  Gain=1/SM.I_nom
  Gain13 : Gain  Gain=1/BUS.Vdc
  Gain14 : Gain  Gain=1/BUS.Idc_nom
  Gain15 : Gain  Gain=1/BUS.Vdc
  Gain17 : Gain  Gain=1/TUG.Tpnom
  Gain18 : Gain  Gain=1/TUG.Fpnom
  Gain19 : Gain  Gain=1/TUG.Vn
  Gain2 : Gain  Gain=1/MOT.Tenom
  Gain20 : Gain  Gain=1/BUS.Idc_nom
  Gain21 : Gain  Gain=1/MOT.Tenom
  Gain23 : Gain  Gain=1/TUG.Fpnom
  Gain28 : Gain  Gain=1/TUG.Vn
  Gain29 : Gain  Gain=MOT.p/MOT.Wnom
  Gain3 : Gain  Gain=1/pi
  Gain30 : Gain  Gain=1/MOT.Pnom
  Gain31 : Gain  Gain=1/MOT.Wmnom
  Gain33 : Gain  Gain=1/MOT.Tenom
  Gain6 : Gain  Gain=1/BAT.V_nom
  Gain7 : Gain  Gain=1/SM.V_nom
  Magnitude-Angle to Complex1 : MagnitudeAngleToComplex  Input=Angle  ConstantPart=1
  Mux{1..2,5,8,10} (5 alike) : Mux  Inputs=2
  Product6 : Product  RndMeth=Zero
  To Workspace : ToWorkspace  VariableName=V_star  SaveFormat=Timeseries  SampleTime=Ts
      settings: Decimation=DF
  To Workspace1 : ToWorkspace  VariableName=mode  SaveFormat=Timeseries  SampleTime=Ts
      settings: Decimation=DF
  To Workspace10 : ToWorkspace  VariableName=Te  SaveFormat=Timeseries  SampleTime=Ts
      settings: Decimation=DF
  To Workspace11 : ToWorkspace  VariableName=wm  SaveFormat=Timeseries  SampleTime=Ts
      settings: Decimation=DF
  To Workspace12 : ToWorkspace  VariableName=Om  SaveFormat=Timeseries  SampleTime=Ts
      settings: Decimation=DF
  To Workspace13 : ToWorkspace  VariableName=iABC  SaveFormat=Timeseries  SampleTime=Ts
      settings: Decimation=DF
  To Workspace14 : ToWorkspace  VariableName=iDEF  SaveFormat=Timeseries  SampleTime=Ts
      settings: Decimation=DF
  To Workspace15 : ToWorkspace  VariableName=idqp  SaveFormat=Timeseries  SampleTime=Ts
      settings: Decimation=DF
  To Workspace16 : ToWorkspace  VariableName=idqpstar  SaveFormat=Timeseries  SampleTime=Ts
      settings: Decimation=DF
  To Workspace17 : ToWorkspace  VariableName=idqm  SaveFormat=Timeseries  SampleTime=Ts
      settings: Decimation=DF
  To Workspace18 : ToWorkspace  VariableName=idqmstar  SaveFormat=Timeseries  SampleTime=Ts
      settings: Decimation=DF
  To Workspace19 : ToWorkspace  VariableName=i0z  SaveFormat=Timeseries  SampleTime=Ts
      settings: Decimation=DF
  To Workspace2 : ToWorkspace  VariableName=wm_star  SaveFormat=Timeseries  SampleTime=Ts
      settings: Decimation=DF
  To Workspace20 : ToWorkspace  VariableName=vBP  SaveFormat=Timeseries  SampleTime=Ts
      settings: Decimation=DF
  To Workspace21 : ToWorkspace  VariableName=iBP  SaveFormat=Timeseries  SampleTime=Ts
      settings: Decimation=DF
  To Workspace22 : ToWorkspace  VariableName=vSM  SaveFormat=Timeseries  SampleTime=Ts
      settings: Decimation=DF
  To Workspace23 : ToWorkspace  VariableName=iSM  SaveFormat=Timeseries  SampleTime=Ts
      settings: Decimation=DF
  To Workspace24 : ToWorkspace  VariableName=vDC_ABC  SaveFormat=Timeseries  SampleTime=Ts
      settings: Decimation=DF
  To Workspace25 : ToWorkspace  VariableName=iDC_ABC  SaveFormat=Timeseries  SampleTime=Ts
      settings: Decimation=DF
  To Workspace26 : ToWorkspace  VariableName=vDC_DEF  SaveFormat=Timeseries  SampleTime=Ts
      settings: Decimation=DF
  To Workspace27 : ToWorkspace  VariableName=iDC_DEF  SaveFormat=Timeseries  SampleTime=Ts
      settings: Decimation=DF
  To Workspace28 : ToWorkspace  VariableName=SoC_BP  SaveFormat=Timeseries  SampleTime=Ts
      settings: Decimation=DF
  To Workspace29 : ToWorkspace  VariableName=SoE_SM  SaveFormat=Timeseries  SampleTime=Ts
      settings: Decimation=DF
  To Workspace3 : ToWorkspace  VariableName=Te_star  SaveFormat=Timeseries  SampleTime=Ts
      settings: Decimation=DF
  To Workspace4 : ToWorkspace  VariableName=DTestar  SaveFormat=Timeseries  SampleTime=Ts
      settings: Decimation=DF
  To Workspace5 : ToWorkspace  VariableName=V  SaveFormat=Timeseries  SampleTime=Ts
      settings: Decimation=DF
  To Workspace6 : ToWorkspace  VariableName=Tp  SaveFormat=Timeseries  SampleTime=Ts
      settings: Decimation=DF
  To Workspace7 : ToWorkspace  VariableName=Ft  SaveFormat=Timeseries  SampleTime=Ts
      settings: Decimation=DF
  To Workspace8 : ToWorkspace  VariableName=Fr  SaveFormat=Timeseries  SampleTime=Ts
      settings: Decimation=DF
  To Workspace9 : ToWorkspace  VariableName=Pe  SaveFormat=Timeseries  SampleTime=Ts
      settings: Decimation=DF
  wires:
  In Bus Element11/1 -> To Workspace29/1  "SoE_SM"
  In Bus Element10/1 -> To Workspace28/1  "SoC_BP"
  Complex to Real-Imag2/1 -> Mux10/1
  [i0z] -> Complex to Real-Imag2/1
  Mux10/1 -> Gain16/1
  Complex to Real-Imag2/2 -> Mux10/2
  Complex to Real-Imag4/1 -> Mux5/1
  Complex to Real-Imag5/2 -> Mux8/2
  [idqm] -> Complex to Real-Imag4/1
  Mux8/1 -> Gain11/1
  Mux5/1 -> Gain9/1
  [idqmstar] -> Complex to Real-Imag5/1
  Complex to Real-Imag5/1 -> Mux8/1
  Complex to Real-Imag4/2 -> Mux5/2
  In Bus Element3/1 -> Gain10/1
  In Bus Element2/1 -> Gain4/1
  Complex to Real-Imag/2 -> Mux1/2
  Complex to Real-Imag1/1 -> Mux2/1
  [idqpstar] -> Complex to Real-Imag1/1
  Mux1/1 -> Gain5/1
  Mux2/1 -> Gain8/1
  [idqp] -> Complex to Real-Imag/1
  Complex to Real-Imag1/2 -> Mux2/2
  Complex to Real-Imag/1 -> Mux1/1
  In Bus Element24/1 -> Gain28/1  "V*"
  Gain28/1 -> To Workspace/1  "V*"
  In Bus Element25/1 -> To Workspace1/1  "mode"
  [wmstar] -> Gain29/1  "wm*"
  Gain29/1 -> To Workspace2/1  "wm*"
  In Bus Element26/1 -> Gain31/1
  Gain31/1 -> To Workspace11/1  "wm"
  [Testar] -> Gain21/1
  [Te] -> Gain33/1
  Gain21/1 -> To Workspace3/1  "Te*"
  Gain33/1 -> To Workspace10/1  "Te"
  [Tp] -> Gain17/1
  Gain17/1 -> To Workspace6/1  "Tp"
  Gain18/1 -> To Workspace7/1  "Ft"
  Gain23/1 -> To Workspace8/1  "Fr"
  In Bus Element20/1 -> Gain19/1  "V"
  Gain19/1 -> To Workspace5/1  "V"
  [Ft] -> Gain18/1  "Ft"
  [Fr] -> Gain23/1  "Fr"
  Gain30/1 -> To Workspace9/1  "Pe"
  In Bus Element22/1 -> Product6/2  "Wm"
  [Te] -> Product6/1  "Te"
  Product6/1 -> Gain30/1  "Pe"
  In Bus Element4/1 -> Gain6/1
  In Bus Element5/1 -> Gain1/1
  In Bus Element6/1 -> Gain7/1
  In Bus Element13/1 -> Gain15/1
  In Bus Element15/1 -> Gain20/1
  In Bus Element14/1 -> Gain14/1
  In Bus Element7/1 -> Gain12/1
  In Bus Element12/1 -> Gain13/1
  Magnitude-Angle to Complex1/1 -> Complex to Magnitude-Angle1/1
  Complex to Magnitude-Angle1/1 -> Gain3/1
  In Bus Element16/1 -> Magnitude-Angle to Complex1/1
  Gain3/1 -> To Workspace12/1  "Om"
  Gain4/1 -> To Workspace13/1
  Gain10/1 -> To Workspace14/1
  Gain8/1 -> To Workspace16/1
  Gain5/1 -> To Workspace15/1
  Gain9/1 -> To Workspace17/1
  Gain11/1 -> To Workspace18/1
  Gain2/1 -> To Workspace4/1  "Te"
  [DTestar] -> Gain2/1
  Gain6/1 -> To Workspace20/1
  Gain1/1 -> To Workspace21/1
  Gain7/1 -> To Workspace22/1
  Gain12/1 -> To Workspace23/1
  Gain13/1 -> To Workspace24/1
  Gain14/1 -> To Workspace25/1
  Gain20/1 -> To Workspace27/1
  Gain15/1 -> To Workspace26/1
  Gain16/1 -> To Workspace19/1

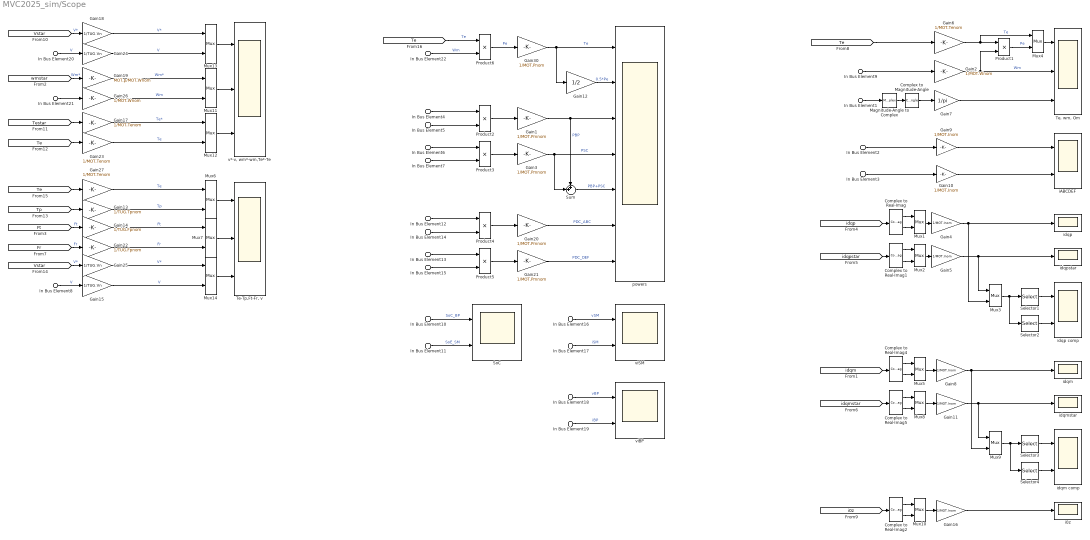
== system MVC2025_sim/Scope ==
  In Bus Element9 : Inport  PortName=DAQ  Element=w
  In Bus Element21 : Inport  PortName=DAQ  Element=w
  In Bus Element1 : Inport  PortName=DAQ  Element=O
  In Bus Element2 : Inport  PortName=DAQ  Element=iABC
  In Bus Element3 : Inport  PortName=DAQ  Element=iDEF
  In Bus Element4 : Inport  PortName=DAQ  Element=vBP
  In Bus Element18 : Inport  PortName=DAQ  Element=vBP
  In Bus Element5 : Inport  PortName=DAQ  Element=iBP
  In Bus Element19 : Inport  PortName=DAQ  Element=iBP
  In Bus Element6 : Inport  PortName=DAQ  Element=vSM
  In Bus Element16 : Inport  PortName=DAQ  Element=vSM
  In Bus Element7 : Inport  PortName=DAQ  Element=iSM
  In Bus Element17 : Inport  PortName=DAQ  Element=iSM
  In Bus Element8 : Inport  PortName=DAQ  Element=V
  In Bus Element20 : Inport  PortName=DAQ  Element=V
  In Bus Element10 : Inport  PortName=DAQ  Element=SoC_BP
  In Bus Element11 : Inport  PortName=DAQ  Element=SoE_SM
  In Bus Element12 : Inport  PortName=DAQ  Element=VDC_ABC
  In Bus Element13 : Inport  PortName=DAQ  Element=VDC_DEF
  In Bus Element14 : Inport  PortName=DAQ  Element=iDC_ABC
  In Bus Element15 : Inport  PortName=DAQ  Element=iDC_DEF
  In Bus Element22 : Inport  PortName=DAQ  Element=wm
  Complex to Real-Imag{,1..2,4..5} (5 alike) : ComplexToRealImag
  Complex to Magnitude-Angle : ComplexToMagnitudeAngle  Output=Angle
  Gain{1,3,20..21} (4 alike) : Gain  Gain=1/MOT.Pmnom
  Gain{4..5,8..11,16} (7 alike) : Gain  Gain=1/MOT.Inom
  Gain12 : Gain  Gain=1/2
  Gain13 : Gain  Gain=1/TUG.Tpnom
  Gain14 : Gain  Gain=1/TUG.Fpnom
  Gain{15,18,24..25} (4 alike) : Gain  Gain=1/TUG.Vn
  Gain{6,17,23,27} (4 alike) : Gain  Gain=1/MOT.Tenom
  Gain19 : Gain  Gain=MOT.p/MOT.Wnom
  Gain2 : Gain  Gain=1/MOT.Wnom
  Gain22 : Gain  Gain=1/TUG.Fpnom
  Gain26 : Gain  Gain=1/MOT.Wnom
  Gain30 : Gain  Gain=1/MOT.Pnom
  Gain7 : Gain  Gain=1/pi
  Magnitude-Angle to Complex : MagnitudeAngleToComplex  Input=Angle  ConstantPart=1
  Mux{1..14} (14 alike) : Mux  Inputs=2
  Product{1..6} (6 alike) : Product  RndMeth=Zero
  Selector1 : Selector  InputPortWidth=4  IndexOptions=Index vector (dialog)  Indices=[1 3]  OutputSizes=1
  Selector2 : Selector  InputPortWidth=4  IndexOptions=Index vector (dialog)  Indices=[2 4]  OutputSizes=1
  Selector3 : Selector  InputPortWidth=4  IndexOptions=Index vector (dialog)  Indices=[1 3]  OutputSizes=1
  Selector4 : Selector  InputPortWidth=4  IndexOptions=Index vector (dialog)  Indices=[2 4]  OutputSizes=1
  SoC : Scope  NumInputPorts=2
  Sum : Sum  Inputs=++|
  "Te, wm, Om" : Scope  NumInputPorts=3
  "Te-Tp,Ft-Fr, v" : Scope  NumInputPorts=3
  i0z : Scope
  iABCDEF : Scope  NumInputPorts=2
  idqm : Scope
  idqm comp : Scope  NumInputPorts=2
  idqmstar : Scope
  idqp : Scope
  idqp comp : Scope  NumInputPorts=2
  idqpstar : Scope
  powers : Scope  NumInputPorts=7
  "v*-v, wm*-wm,Te*-Te" : Scope  NumInputPorts=3
  viBP : Scope  NumInputPorts=2
  viSM : Scope  NumInputPorts=2
  wires:
  In Bus Element9/1 -> Gain2/1
  Gain7/1 -> "Te, wm, Om"/3
  Complex to Real-Imag/1 -> Mux1/1
  Complex to Real-Imag1/2 -> Mux2/2
  Magnitude-Angle to Complex/1 -> Complex to Magnitude-Angle/1
  Selector2/1 -> idqp comp/2
  [Te] -> Gain6/1
  [idqp] -> Complex to Real-Imag/1
  Selector1/1 -> idqp comp/1
  Complex to Magnitude-Angle/1 -> Gain7/1
  Mux4/1 -> "Te, wm, Om"/1
  Gain2/1 -> "Te, wm, Om"/2, Product1/2  "Wm"
  Mux2/1 -> Gain5/1
  Gain5/1 -> idqpstar/1, Mux3/1
  Gain4/1 -> idqp/1, Mux3/2
  Mux1/1 -> Gain4/1
  Gain6/1 -> Product1/1, Mux4/1  "Te"
  [idqpstar] -> Complex to Real-Imag1/1
  Complex to Real-Imag1/1 -> Mux2/1
  Mux3/1 -> Selector1/1, Selector2/1
  Complex to Real-Imag/2 -> Mux1/2
  In Bus Element2/1 -> Gain9/1
  In Bus Element3/1 -> Gain10/1
  Gain9/1 -> iABCDEF/1
  Gain10/1 -> iABCDEF/2
  In Bus Element1/1 -> Magnitude-Angle to Complex/1
  Complex to Real-Imag4/2 -> Mux5/2
  Mux9/1 -> Selector4/1, Selector3/1
  Complex to Real-Imag5/1 -> Mux8/1
  [idqmstar] -> Complex to Real-Imag5/1
  Mux5/1 -> Gain8/1
  Gain8/1 -> idqm/1, Mux9/2
  Gain11/1 -> idqmstar/1, Mux9/1
  Mux8/1 -> Gain11/1
  Selector3/1 -> idqm comp/1
  [idqm] -> Complex to Real-Imag4/1
  Selector4/1 -> idqm comp/2
  Complex to Real-Imag5/2 -> Mux8/2
  Complex to Real-Imag4/1 -> Mux5/1
  In Bus Element5/1 -> Product2/2
  In Bus Element4/1 -> Product2/1
  Product2/1 -> Gain1/1
  Gain1/1 -> Sum/1, powers/3  "PBP"
  Gain3/1 -> Sum/2, powers/4  "PSC"
  Product3/1 -> Gain3/1
  In Bus Element6/1 -> Product3/1
  In Bus Element7/1 -> Product3/2
  Gain12/1 -> powers/2  "0.5*Pe"
  [Tp] -> Gain13/1
  Gain13/1 -> Mux6/2  "Tp"
  Mux6/1 -> "Te-Tp,Ft-Fr, v"/1
  Gain14/1 -> Mux7/1  "Ft"
  Gain22/1 -> Mux7/2  "Fr"
  Mux7/1 -> "Te-Tp,Ft-Fr, v"/2
  In Bus Element8/1 -> Gain15/1  "V"
  Gain15/1 -> Mux14/2  "V"
  Complex to Real-Imag2/2 -> Mux10/2
  Mux10/1 -> Gain16/1
  Gain16/1 -> i0z/1
  [i0z] -> Complex to Real-Imag2/1
  Complex to Real-Imag2/1 -> Mux10/1
  [Testar] -> Gain17/1
  [Te] -> Gain23/1
  Mux12/1 -> "v*-v, wm*-wm,Te*-Te"/3
  [wmstar] -> Gain19/1  "Wm*"
  Gain18/1 -> Mux13/1  "V*"
  Mux13/1 -> "v*-v, wm*-wm,Te*-Te"/1
  Mux11/1 -> "v*-v, wm*-wm,Te*-Te"/2
  Gain19/1 -> Mux11/1  "Wm*"
  In Bus Element10/1 -> SoC/1  "SoC_BP"
  In Bus Element11/1 -> SoC/2  "SoE_SM"
  In Bus Element12/1 -> Product4/1
  In Bus Element14/1 -> Product4/2
  In Bus Element13/1 -> Product5/1
  In Bus Element15/1 -> Product5/2
  Product4/1 -> Gain20/1
  Product5/1 -> Gain21/1
  Gain20/1 -> powers/6  "PDC_ABC"
  Gain21/1 -> powers/7  "PDC_DEF"
  Sum/1 -> powers/5  "PBP+PSC"
  [Ft] -> Gain14/1  "Ft"
  [Fr] -> Gain22/1  "Fr"
  [Vstar] -> Gain18/1  "V*"
  Gain17/1 -> Mux12/1  "Te*"
  Gain23/1 -> Mux12/2  "Te"
  Mux14/1 -> "Te-Tp,Ft-Fr, v"/3
  In Bus Element16/1 -> viSM/1  "vSM"
  In Bus Element17/1 -> viSM/2  "iSM"
  In Bus Element18/1 -> viBP/1  "vBP"
  In Bus Element19/1 -> viBP/2  "iBP"
  In Bus Element20/1 -> Gain24/1  "V"
  Gain24/1 -> Mux13/2  "V"
  [Vstar] -> Gain25/1  "V*"
  Gain25/1 -> Mux14/1  "V*"
  In Bus Element21/1 -> Gain26/1
  Gain26/1 -> Mux11/2  "Wm"
  [Te] -> Gain27/1
  Gain27/1 -> Mux6/1  "Te"
  [Te] -> Product6/1  "Te"
  In Bus Element22/1 -> Product6/2  "Wm"
  Product6/1 -> Gain30/1  "Pe"
  Product1/1 -> Mux4/2  "Pe"
  Gain30/1 -> Gain12/1, powers/1  "Te"
